simulink model "gotoPointDiff"  (Simulink 8.3)
settings: Solver=ode45  StartTime=0.0  StopTime=10  RelTol=1e-3
undefined symbols (not defined in the file): l, r, x0, xg
libraries: simulink x2
settings Model: Creator=dariush  LastModifiedBy=dariush
settings DataIOCC: SignalLoggingSaveFormat=Dataset
settings DebuggingCC: UnderspecifiedInitializationDetection=Simplified  StateNameClashWarn=none
settings GRTTargetCC: CombineOutputUpdateFcns=on  GRTInterface=off

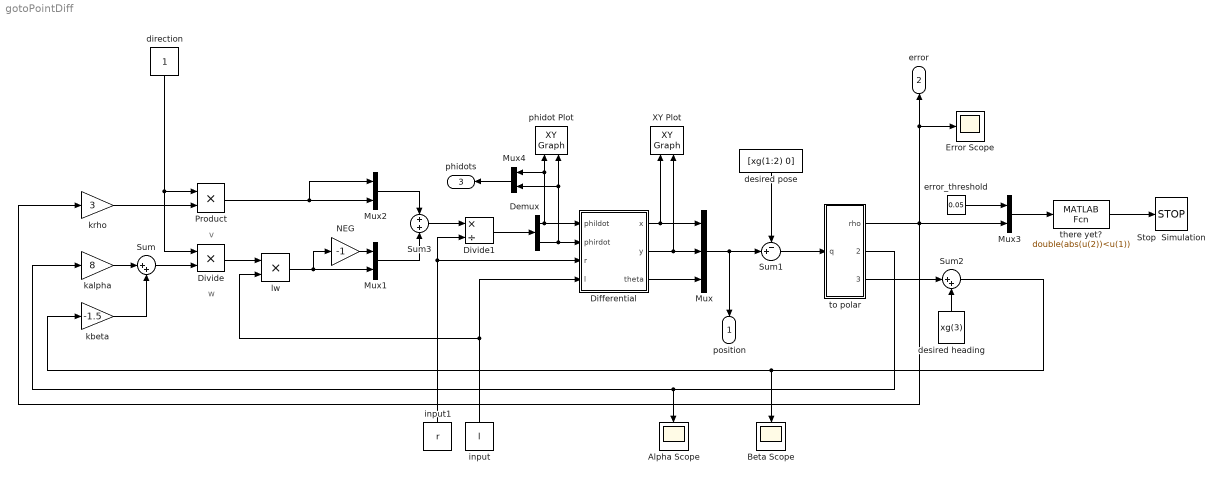
== system gotoPointDiff ==
  note: w
  note: v
  Alpha Scope : Scope
      settings: SaveName=ScopeData2
  Beta Scope : Scope
  Demux : Demux  Outputs=2
  Differential : Subsystem  mask{x0=x0}
      mask prompts: x0 "Initial States"
  Divide : Product  Inputs=**  RndMeth=Zero
  Divide1 : Product  Inputs=*/  RndMeth=Round
  Error Scope : Scope
  Mux : Mux  Inputs=3
  Mux{1..4} (4 alike) : Mux  Inputs=2
  NEG : Gain  Gain=-1
  Product : Product  RndMeth=Zero
  Stop  Simulation : Stop
  Sum : Sum  Inputs=|++
  Sum1 : Sum  Inputs=-+|
  Sum2 : Sum  Inputs=|++
  Sum3 : Sum  Inputs=+|+
  XY Plot : simulink/Sinks/XY Graph  xmin=-15  xmax=15  ymin=-15  ymax=15  st=-1
  desired heading : Constant  Value=xg(3)
  desired pose : Constant  Value=[xg(1:2) 0]
  direction : Constant
  error_threshold : Constant  Value=0.05
  input : Constant  Value=l
  input1 : Constant  Value=r
  kalpha : Gain  Gain=8
  kbeta : Gain  Gain=-1.5
  krho : Gain  Gain=3
  lw : Product
  phidot Plot : simulink/Sinks/XY Graph  xmin=-15  xmax=15  ymin=-15  ymax=15  st=-1
  there yet? : MATLABFcn  MATLABFcn=double(abs(u(2))<u(1))  OutputSignalType=real
  to polar : Subsystem
  position : Outport
  error : Outport  Port=2
  phidots : Outport  Port=3
  wires:
  Differential/1(x) -> XY Plot/1, Mux/1
  Differential/2(y) -> XY Plot/2, Mux/2
  Mux/1 -> Sum1/2, position/1
  desired pose/1 -> Sum1/1
  Sum1/1 -> to polar/1(q)
  there yet?/1 -> Stop  Simulation/1
  to polar/3(beta) -> Sum2/1
  desired heading/1 -> Sum2/2
  Sum2/1 -> Beta Scope/1, kbeta/1
  to polar/2(alpha) -> Alpha Scope/1, kalpha/1
  kalpha/1 -> Sum/1
  kbeta/1 -> Sum/2
  Sum/1 -> Divide/2
  krho/1 -> Product/2
  Divide/1 -> lw/1
  input/1 -> Differential/4(l), lw/2
  input1/1 -> Differential/3(r), Divide1/2
  lw/1 -> NEG/1, Mux1/2
  NEG/1 -> Mux1/1
  Product/1 -> Mux2/1, Mux2/2
  Mux1/1 -> Sum3/2
  Mux2/1 -> Sum3/1
  Sum3/1 -> Divide1/1
  Demux/1 -> phidot Plot/1, Mux4/1, Differential/1(phildot)
  Demux/2 -> phidot Plot/2, Mux4/2, Differential/2(phirdot)
  to polar/1(rho) -> error/1, Error Scope/1, Mux3/2, krho/1
  error_threshold/1 -> Mux3/1
  Mux3/1 -> there yet?/1
  Differential/3(theta) -> Mux/3
  Mux4/1 -> phidots/1
  Divide1/1 -> Demux/1
  direction/1 -> Divide/1, Product/1

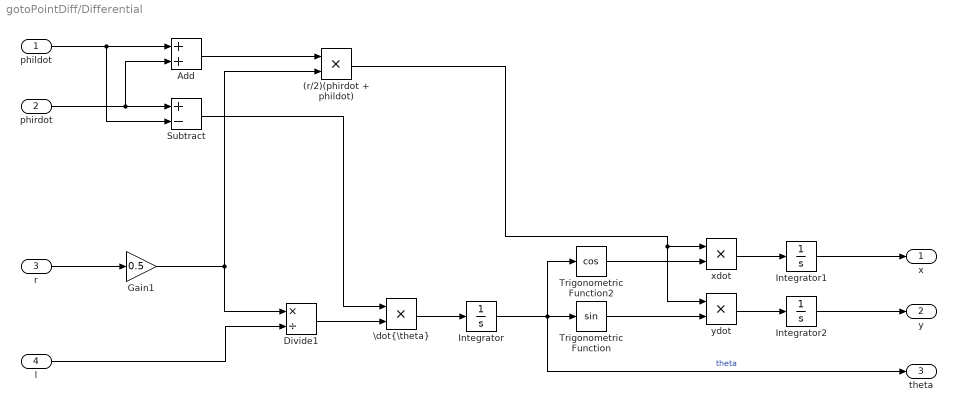
== system gotoPointDiff/Differential ==
  phildot : Inport
  phirdot : Inport  Port=2
  r : Inport  Port=3
  l : Inport  Port=4
  (r/2)(phirdot + phildot) : Product
  Add : Sum
  Divide1 : Product  Inputs=*/
  Gain1 : Gain  Gain=0.5
  Integrator : Integrator  InitialCondition=x0(3)
  Integrator1 : Integrator  InitialCondition=x0(1)
  Integrator2 : Integrator  InitialCondition=x0(2)
  Subtract : Sum  Inputs=+-
  Trigonometric Function : Trigonometry
  Trigonometric Function2 : Trigonometry  Operator=cos
  "\\dot{\\theta}" : Product
  xdot : Product
  ydot : Product
  x : Outport
  y : Outport  Port=2
  theta : Outport  Port=3
  wires:
  Subtract/1 -> "\\dot{\\theta}"/1
  l/1 -> Divide1/2
  Trigonometric Function/1 -> ydot/2
  Integrator/1 -> theta/1, Trigonometric Function/1, Trigonometric Function2/1  "theta"
  (r/2)(phirdot + phildot)/1 -> ydot/1, xdot/1
  Divide1/1 -> "\\dot{\\theta}"/2
  phirdot/1 -> Add/2, Subtract/1
  Integrator2/1 -> y/1
  Integrator1/1 -> x/1
  "\\dot{\\theta}"/1 -> Integrator/1
  r/1 -> Gain1/1
  phildot/1 -> Subtract/2, Add/1
  ydot/1 -> Integrator2/1
  Trigonometric Function2/1 -> xdot/2
  xdot/1 -> Integrator1/1
  Gain1/1 -> Divide1/1, (r/2)(phirdot + phildot)/2
  Add/1 -> (r/2)(phirdot + phildot)/1

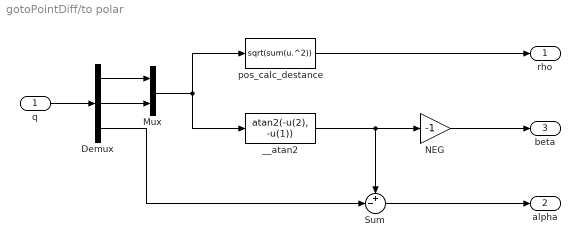
== system gotoPointDiff/to polar ==
  q : Inport
  Demux : Demux  Outputs=3
  Mux : Mux  Inputs=2
  NEG : Gain  Gain=-1
  Sum : Sum  Inputs=+-|
  __atan2 : MATLABFcn  MATLABFcn=atan2(-u(2), -u(1))  OutputDimensions=1
  pos_calc_destance : MATLABFcn  MATLABFcn=sqrt(sum(u.^2))  OutputDimensions=1
  rho : Outport
  alpha : Outport  Port=2
  beta : Outport  Port=3
  wires:
  NEG/1 -> beta/1
  q/1 -> Demux/1
  pos_calc_destance/1 -> rho/1
  Demux/1 -> Mux/1
  Mux/1 -> pos_calc_destance/1, __atan2/1
  Demux/2 -> Mux/2
  __atan2/1 -> NEG/1, Sum/1
  Demux/3 -> Sum/2
  Sum/1 -> alpha/1
